simulink model "Discrete_PID_model_3_2_2"  (R2024b)
settings: Solver=ode5  StartTime=0.0  StopTime=20  FixedStep=0.001  RelTol=1e-3
undefined symbols (not defined in the file): DiscIntNeverNeededParam, Gam_o, H_o, J_o, K, ki, National_Instruments, Nu, Nx, PCI, Phi_o, rpm2rads, sens, step_gain, T, u_bar_max
libraries: sldrtlib x3
settings Model: SimulationMode=external  ExtModeTrigDuration=20001  Creator=fasoloandr  LastModifiedBy=Enrico
settings DataIOCC: ReturnWorkspaceOutputs=off
settings HardwareCC: ProdBitPerLong=64  ProdHWDeviceType=Intel->x86-64 (Linux 64)
settings RTWCC: Description=Simulink Desktop Real-Time  SystemTargetFile=sldrt.tlc  TemplateMakefile=sldrt.tmf  RTWCompilerOptimization=on
settings CodeAppCC: MaxIdLength=95
settings SimulinkDesktopRealTimeCC: TargetLibSuffix=_sldrt.a  TargetPreCompLibLocation=D:\Programmi (D)\MATLAB\R2024b\toolbox\sldrt\lib\win64  ParMdlRefBuildCompliant=on

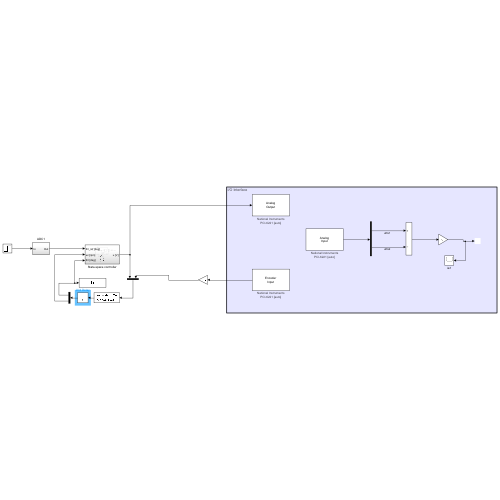
[thumbnail: Simulink's stored preview of the top-level diagram]
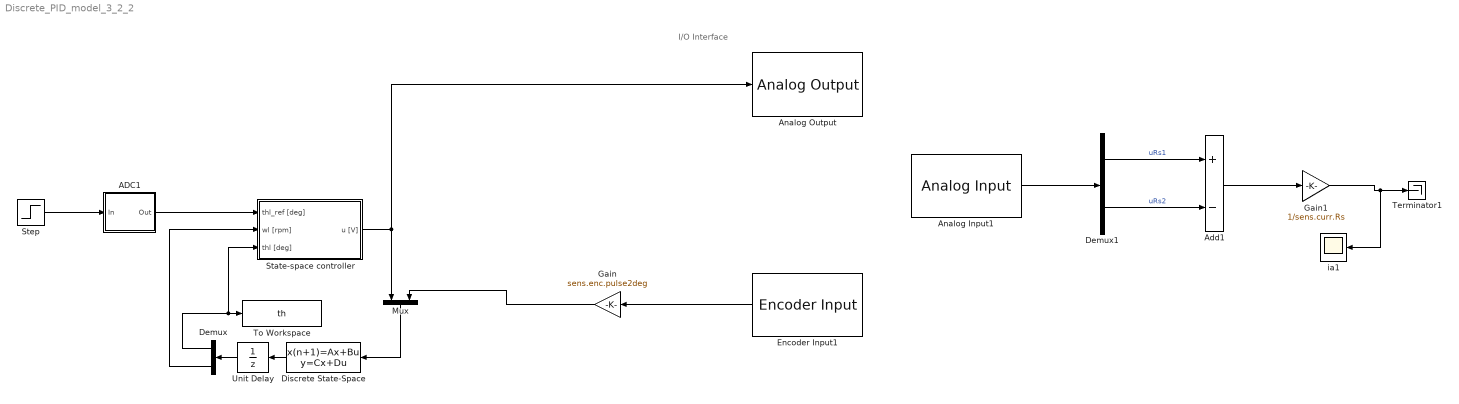
== system Discrete_PID_model_3_2_2 ==
  note: I/O Interface
  ADC1 : Subsystem
  Add1 : Sum  Inputs=+-
  Analog Input1 : sldrtlib/Analog Input  SampleTime=-1  MaxMissedTicks=10  ShowMissedTicks=off  YieldWhenWaiting=off  DrvName=National_Instruments/PCI-6221  DrvAddress=4294967295  DrvOptions=[0 0 0 2 0]  Channels=[1,2]  RangeMode=1  VoltRange=1  DataType=1
      settings: AttributesFormatString=National Instruments\nPCI-6221 [auto]
  Analog Output : sldrtlib/Analog Output  SampleTime=-1  MaxMissedTicks=10  ShowMissedTicks=off  YieldWhenWaiting=off  DrvName=National_Instruments/PCI-6221  DrvAddress=4294967295  DrvOptions=[0 0 0 2 0]  Channels=1  RangeMode=1  VoltRange=1  InitialValue=[0]  FinalValue=[0]
      settings: AttributesFormatString=National Instruments\nPCI-6221 [auto]
  Demux : Demux  Outputs=2
  Demux1 : Demux  Outputs=2
  Discrete State-Space : DiscreteStateSpace  A=Phi_o  B=Gam_o  C=H_o  D=J_o  SampleTime=T
  Encoder Input1 : sldrtlib/Encoder Input  SampleTime=-1  MaxMissedTicks=10  ShowMissedTicks=off  YieldWhenWaiting=off  DrvName=National_Instruments/PCI-6221  DrvAddress=4294967295  DrvOptions=[0 0 0 2 0]  Channels=1  QuadMode=3  IndexPulse=1  InputFilter=Inf  DataType=1
      settings: AttributesFormatString=National Instruments\nPCI-6221 [auto]
  Gain : Gain  Gain=sens.enc.pulse2deg
  Gain1 : Gain  Gain=1/sens.curr.Rs
  Mux : Mux  Inputs=2
  State-space controller : Subsystem
  Step : Step  After=step_gain  SampleTime=0
  Terminator1 : Terminator
  To Workspace : ToWorkspace  VariableName=th  SaveFormat=Structure With Time  SampleTime=-1
  Unit Delay : UnitDelay  SampleTime=T  HasFrameUpgradeWarning=on
  ia1 : Scope
  wires:
  Gain1/1 -> ia1/1, Terminator1/1
  Demux1/1 -> Add1/1  "uRs1"
  Analog Input1/1 -> Demux1/1
  Demux1/2 -> Add1/2  "uRs2"
  Encoder Input1/1 -> Gain/1
  Add1/1 -> Gain1/1
  ADC1/1(Out) -> State-space controller/1(thl_ref [deg])
  Demux/1 -> State-space controller/3(thl [deg]), To Workspace/1
  Step/1 -> ADC1/1(In)
  Mux/1 -> Discrete State-Space/1
  Gain/1 -> Mux/2
  Demux/2 -> State-space controller/2(wl [rpm])
  State-space controller/1(u [V]) -> Analog Output/1, Mux/1
  Unit Delay/1 -> Demux/1
  Discrete State-Space/1 -> Unit Delay/1

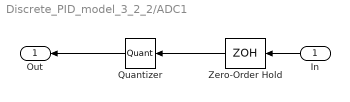
== system Discrete_PID_model_3_2_2/ADC1 ==
  In : Inport
  Quantizer : Quantizer  QuantizationInterval=daq.adc.q
  Zero-Order Hold : ZeroOrderHold  SampleTime=T
  Out : Outport
  wires:
  Quantizer/1 -> Out/1
  In/1 -> Zero-Order Hold/1
  Zero-Order Hold/1 -> Quantizer/1

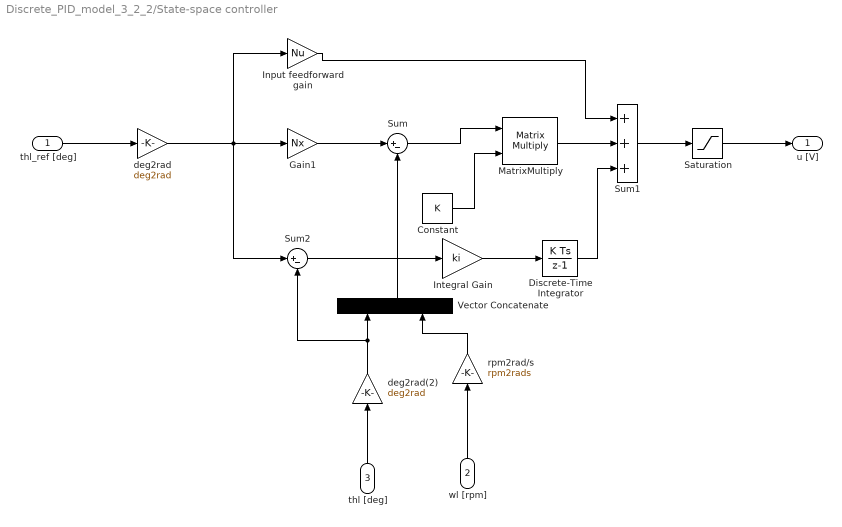
== system Discrete_PID_model_3_2_2/State-space controller ==
  thl_ref [deg] : Inport
  wl [rpm] : Inport  Port=2
  thl [deg] : Inport  Port=3
  Constant : Constant  Value=K
  Discrete-Time Integrator : DiscreteIntegrator  SampleTime=T  ICPrevOutput=DiscIntNeverNeededParam  ICPrevScaledInput=DiscIntNeverNeededParam
  Gain1 : Gain  Gain=Nx
  Input feedforward gain : Gain  Gain=Nu
  Integral Gain : Gain  Gain=ki
  MatrixMultiply : Product  Multiplication=Matrix(*)
  Saturation : Saturate  UpperLimit=u_bar_max  LowerLimit=-u_bar_max
  Sum : Sum  Inputs=|+-
  Sum1 : Sum  Inputs=+++
  Sum2 : Sum  Inputs=|+-
  Vector Concatenate : Concatenate
  deg2rad : Gain  Gain=deg2rad
  deg2rad(2) : Gain  Gain=deg2rad
  rpm2rad/s : Gain  Gain=rpm2rads
  u [V] : Outport
  wires:
  deg2rad(2)/1 -> Vector Concatenate/1, Sum2/2
  Constant/1 -> MatrixMultiply/2
  thl_ref [deg]/1 -> deg2rad/1
  Input feedforward gain/1 -> Sum1/1
  Saturation/1 -> u [V]/1
  MatrixMultiply/1 -> Sum1/2
  Sum/1 -> MatrixMultiply/1
  wl [rpm]/1 -> rpm2rad/s/1
  Vector Concatenate/1 -> Sum/2
  thl [deg]/1 -> deg2rad(2)/1
  deg2rad/1 -> Gain1/1, Sum2/1, Input feedforward gain/1
  rpm2rad/s/1 -> Vector Concatenate/2
  Gain1/1 -> Sum/1
  Sum1/1 -> Saturation/1
  Integral Gain/1 -> Discrete-Time Integrator/1
  Sum2/1 -> Integral Gain/1
  Discrete-Time Integrator/1 -> Sum1/3
